simulink model "AC_base_1_VSM_1_22a"  (R2022a)
settings: Solver=ode3  StartTime=0.0  StopTime=8  FixedStep=HWSampleTime  RelTol=1e-3
undefined symbols (not defined in the file): ControlSampleTime, DiscIntNeverNeededParam, HWSampleTime, Ipwm_back, Ipwm_off, LCL, Manage, Oversample, Param, scaling_factor, SM, Ts, V_DC, VSMCTRL
libraries: fl_lib x51, nesl_utility x35, simulink x19, FriedrichLibrary x19, ee_lib x14, simulink_extras x7, TriphaseHardwaremodule x6, spsPower3phInstantaneousLib x1, spsEdgeDetectorLib x1, StateMachines x1, slpidlib x1
(part 1 of 4)
settings Model: Creator=e2n051  LastModifiedBy=e2n051

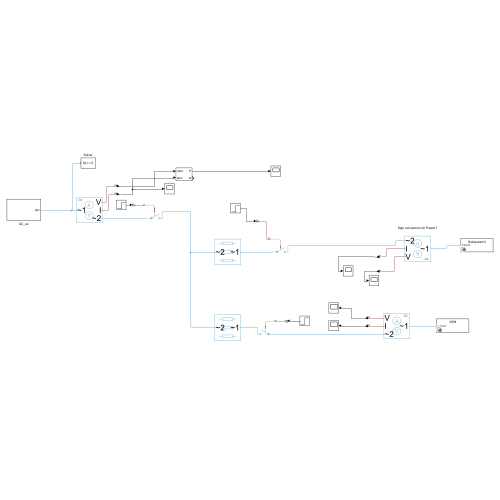
[thumbnail: Simulink's stored preview of the top-level diagram]
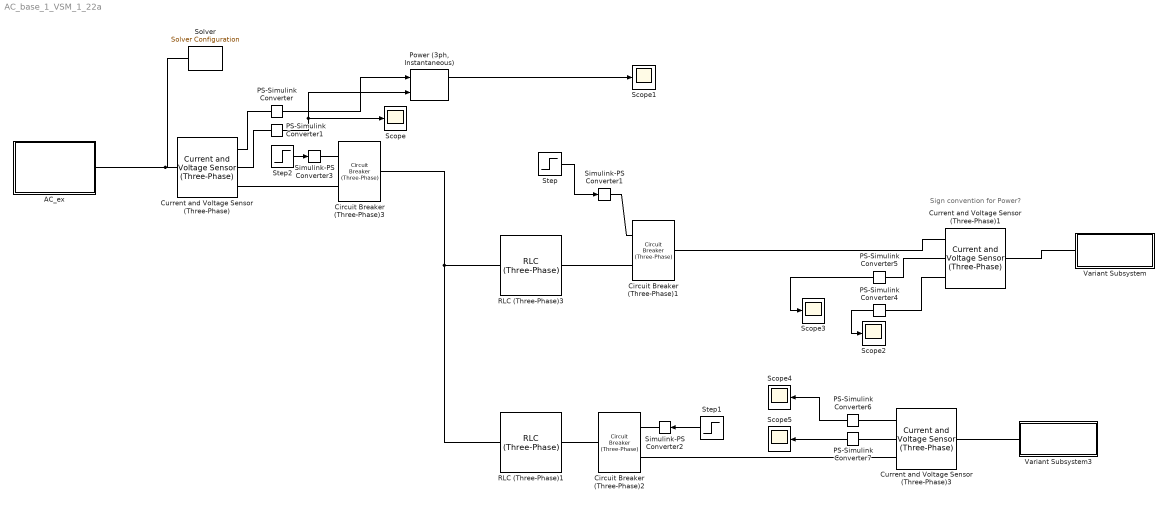
== system AC_base_1_VSM_1_22a ==
  note: Sign convention for Power?
  AC_ex : Subsystem
  Circuit Breaker (Three-Phase)1 : ee_lib/Switches & Breakers/Circuit Breaker (Three-Phase)  R_closed=0.001 Ohm  G_open=1e-6 1/Ohm  threshold=0.5 V  breaker_behavior=ee.enum.switches.breakerBehavior.zeroCrossingEnable
      settings: InternalSimscapePortConfiguration="{\"Bottom\":[],\"Left\":[{\"id\":\"vT\",\"label\":\"vT\",\"type\":\"input\"},{\"id\":\"N1\",\"label\":\"~1\",\"type\":\"foundation.electrical.three_phase\"}],\"Right\":[{\"id\":\"N2\",\"label\":\"~2\",\"type\":\"foundation.electrical.three_phase\"}],\"Top\":[]}"
  Circuit Breaker (Three-Phase)2 : ee_lib/Switches & Breakers/Circuit Breaker (Three-Phase)  R_closed=0.001 Ohm  G_open=1e-6 1/Ohm  threshold=0.5 V  breaker_behavior=ee.enum.switches.breakerBehavior.zeroCrossingEnable
      settings: InternalSimscapePortConfiguration="{\"Bottom\":[],\"Left\":[{\"id\":\"vT\",\"label\":\"vT\",\"type\":\"input\"},{\"id\":\"N1\",\"label\":\"~1\",\"type\":\"foundation.electrical.three_phase\"}],\"Right\":[{\"id\":\"N2\",\"label\":\"~2\",\"type\":\"foundation.electrical.three_phase\"}],\"Top\":[]}"
  Circuit Breaker (Three-Phase)3 : ee_lib/Switches & Breakers/Circuit Breaker (Three-Phase)  R_closed=0.001 Ohm  G_open=1e-6 1/Ohm  threshold=0.5 V  breaker_behavior=ee.enum.switches.breakerBehavior.zeroCrossingEnable
      settings: InternalSimscapePortConfiguration="{\"Bottom\":[],\"Left\":[{\"id\":\"vT\",\"label\":\"vT\",\"type\":\"input\"},{\"id\":\"N1\",\"label\":\"~1\",\"type\":\"foundation.electrical.three_phase\"}],\"Right\":[{\"id\":\"N2\",\"label\":\"~2\",\"type\":\"foundation.electrical.three_phase\"}],\"Top\":[]}"
  Current and Voltage Sensor (Three-Phase) : ee_lib/Sensors & Transducers/Current and Voltage Sensor (Three-Phase)  vMeasurementType=ee.enum.vmeasurement.lg  outputUnit=ee.enum.unit.si  SRated=100e6 A*V  VRated=24e3 V  I_specify=off  I_priority=None  I=[0, 0, 0] A  I_nominal_specify=off  I_nominal_value=1  I_nominal_unit=A  V_specify=off  V_priority=None  V=[0, 0, 0] V  V_nominal_specify=off  V_nominal_value=1  V_nominal_unit=V
      settings: InternalSimscapePortConfiguration="{\"Bottom\":[],\"Left\":[{\"id\":\"N1\",\"label\":\"~1\",\"type\":\"foundation.electrical.three_phase\"}],\"Right\":[{\"id\":\"V_output\",\"label\":\"V\",\"type\":\"output\"},{\"id\":\"I_output\",\"label\":\"I\",\"type\":\"output\"},{\"id\":\"N2\",\"label\":\"~2\",\"type\":\"foundation.electrical.three_phase\"}],\"Top\":[]}"
  Current and Voltage Sensor (Three-Phase)1 : ee_lib/Sensors & Transducers/Current and Voltage Sensor (Three-Phase)  vMeasurementType=ee.enum.vmeasurement.lg  outputUnit=ee.enum.unit.si  SRated=100e6 A*V  VRated=24e3 V  I_specify=off  I_priority=None  I=[0, 0, 0] A  I_nominal_specify=off  I_nominal_value=1  I_nominal_unit=A  V_specify=off  V_priority=None  V=[0, 0, 0] V  V_nominal_specify=off  V_nominal_value=1  V_nominal_unit=V
      settings: InternalSimscapePortConfiguration="{\"Bottom\":[],\"Left\":[{\"id\":\"N1\",\"label\":\"~1\",\"type\":\"foundation.electrical.three_phase\"}],\"Right\":[{\"id\":\"V_output\",\"label\":\"V\",\"type\":\"output\"},{\"id\":\"I_output\",\"label\":\"I\",\"type\":\"output\"},{\"id\":\"N2\",\"label\":\"~2\",\"type\":\"foundation.electrical.three_phase\"}],\"Top\":[]}"
  Current and Voltage Sensor (Three-Phase)3 : ee_lib/Sensors & Transducers/Current and Voltage Sensor (Three-Phase)  vMeasurementType=ee.enum.vmeasurement.lg  outputUnit=ee.enum.unit.si  SRated=100e6 A*V  VRated=24e3 V  I_specify=off  I_priority=None  I=[0, 0, 0] A  I_nominal_specify=off  I_nominal_value=1  I_nominal_unit=A  V_specify=off  V_priority=None  V=[0, 0, 0] V  V_nominal_specify=off  V_nominal_value=1  V_nominal_unit=V
      settings: InternalSimscapePortConfiguration="{\"Bottom\":[],\"Left\":[{\"id\":\"N1\",\"label\":\"~1\",\"type\":\"foundation.electrical.three_phase\"}],\"Right\":[{\"id\":\"V_output\",\"label\":\"V\",\"type\":\"output\"},{\"id\":\"I_output\",\"label\":\"I\",\"type\":\"output\"},{\"id\":\"N2\",\"label\":\"~2\",\"type\":\"foundation.electrical.three_phase\"}],\"Top\":[]}"
  PS-Simulink Converter{,1,4..7} (6 alike) : nesl_utility/PS-Simulink Converter  PhysicalDomain=network_engine_domain  SubClassName=ps_output  LeftPortType=input  RightPortType=output  PseudoPeriodic=off  Frequencies=[]  VectorFormat=inherit  Unit=inherit  AffineConversion=off
  "Power (3ph, Instantaneous)" : spsPower3phInstantaneousLib/Power (3ph, Instantaneous)
  RLC (Three-Phase)1 : ee_lib/Passive/RLC Assemblies/RLC (Three-Phase)  port_option=ee.enum.threePhasePort.composite  component_structure=ee.enum.rlc.structure.R  R=0.1 Ohm  L=1e-2 H  C=1e-6 F  R_parasitic=0 Ohm  G_parasitic=0 1/Ohm  IL_specify=off  IL_priority=High  IL=[0, 0, 0] A  IL_nominal_specify=off  IL_nominal_value=1  IL_nominal_unit=A  VC_specify=off  VC_priority=High  VC=[0, 0, 0] V  VC_nominal_specify=off  VC_nominal_value=1  VC_nominal_unit=V
      settings: InternalSimscapePortConfiguration="{\"Bottom\":[],\"Left\":[{\"id\":\"N1\",\"label\":\"~1\",\"type\":\"foundation.electrical.three_phase\"}],\"Right\":[{\"id\":\"N2\",\"label\":\"~2\",\"type\":\"foundation.electrical.three_phase\"}],\"Top\":[]}"
  RLC (Three-Phase)3 : ee_lib/Passive/RLC Assemblies/RLC (Three-Phase)  port_option=ee.enum.threePhasePort.composite  component_structure=ee.enum.rlc.structure.R  R=1 Ohm  L=1e-2 H  C=1e-6 F  R_parasitic=0 Ohm  G_parasitic=0 1/Ohm  IL_specify=off  IL_priority=High  IL=[0, 0, 0] A  IL_nominal_specify=off  IL_nominal_value=1  IL_nominal_unit=A  VC_specify=off  VC_priority=High  VC=[0, 0, 0] V  VC_nominal_specify=off  VC_nominal_value=1  VC_nominal_unit=V
      settings: InternalSimscapePortConfiguration="{\"Bottom\":[],\"Left\":[{\"id\":\"N1\",\"label\":\"~1\",\"type\":\"foundation.electrical.three_phase\"}],\"Right\":[{\"id\":\"N2\",\"label\":\"~2\",\"type\":\"foundation.electrical.three_phase\"}],\"Top\":[]}"
  Scope{,1..5} (6 alike) : Scope
  Simulink-PS Converter1 : nesl_utility/Simulink-PS Converter  PhysicalDomain=network_engine_domain  SubClassName=ps_input  LeftPortType=input  RightPortType=output  PseudoPeriodic=off  Frequencies=[]  NoiseDistribution=none  NoiseParameters=[]  Unit=1  AffineConversion=off  FilteringAndDerivatives=provide  SimscapeFilterOrder=1  InputFilterTimeConstant=0.001  UdotUserProvided=0
  Simulink-PS Converter2 : nesl_utility/Simulink-PS Converter  PhysicalDomain=network_engine_domain  SubClassName=ps_input  LeftPortType=input  RightPortType=output  PseudoPeriodic=off  Frequencies=[]  NoiseDistribution=none  NoiseParameters=[]  Unit=1  AffineConversion=off  FilteringAndDerivatives=provide  SimscapeFilterOrder=1  InputFilterTimeConstant=0.001  UdotUserProvided=0
  Simulink-PS Converter3 : nesl_utility/Simulink-PS Converter  PhysicalDomain=network_engine_domain  SubClassName=ps_input  LeftPortType=input  RightPortType=output  PseudoPeriodic=off  Frequencies=[]  NoiseDistribution=none  NoiseParameters=[]  Unit=1  AffineConversion=off  FilteringAndDerivatives=provide  SimscapeFilterOrder=1  InputFilterTimeConstant=0.001  UdotUserProvided=0
  Solver : nesl_utility/Solver Configuration  PhysicalDomain=network_engine_domain  SubClassName=solver  LeftPortType=input  RightPortType=generic  Tones=[]  Harmonics=[]  SimulateNoise=off  Profile=off  UseLocalSampling=off  EnableSwitchedLinearOptims=on  FrequencyDomain=off  UseCCode=off  RelTol=0.001  AbsTol=1e-06  MinStep=1e-09  ToWorkspace=off  RevertToSquareIcSolve=off  NumHomotopyIterations=100  PhasorMode=off  PhasorModeNumHarmonics=1  ConsistencySolver=NEWTON_FTOL  IndexReductionMethod=DerivativeReplacement  DoDC=off  ResidualTolerance=1e-2  ConsistencyTolSource=GLOBAL  ConsistencyAbsTol=0.001  ConsistencyRelTol=0.001  ConsistencyTolFactor=0.001  UseLocalSolver=on  LocalSolverChoice=NE_BACKWARD_EULER_ADVANCER  ResolveIndetEquations=on  FunctionEvalNumThread=1  LocalSolverSampleTime=HWSampleTime  DoFixedCost=off  MaxNonlinIter=3  MaxModeIter=2  ComputeImpulses=off  ImpulseIterations=2  LinearAlgebra=Sparse  LinearAlgebraNumThread=0  EquationFormulation=NE_TIME_EF  DelaysMemoryBudget=1024  AutomaticFiltering=on  FilteringTimeConstant=0.001  PartitionStorageMethod=AS_NEEDED  PartitionMemoryBudget=1024  PartitionMethod=FAST  MultibodyUseLocalSolver=off  MultibodyLocalSolverChoice=ODE1  MultibodyLocalSolverSampleTime=0.001
  Step : Step  After=0  SampleTime=0
  Step1 : Step  Time=0  After=0  SampleTime=0
  Step2 : Step  Time=6  SampleTime=0
  Variant Subsystem : Subsystem  Variant=on  VariantControlMode=label  LabelModeActiveChoice=Variant2  mask{VChoice=V2}
      mask prompts: VChoice "Select suystem"
      mask init:
      | choice = get_param(gcb,'VChoice');
      | vssBlk = gcb;
      | oldVariant = get_param(gcb,'LabelModeActiveChoice');
      | if strcmp(choice,'V1')
      |     
      |     set_param(vssBlk, 'LabelModeActiveChoice', 'Variant1');
      | else
      |     
      |     set_param(vssBlk, 'LabelModeActiveChoice', 'Variant2');
      | end
      mask TypeOptions VChoice: V1 | V2
  Variant Subsystem3 : Subsystem  Variant=on  VariantControlMode=label  LabelModeActiveChoice=Variant1  mask{VChoice=VSM}
      mask prompts: VChoice "Select suystem"
      mask init:
      | choice = get_param(gcb,'VChoice');
      | vssBlk = gcb;
      | oldVariant = get_param(gcb,'LabelModeActiveChoice');
      | if strcmp(choice,'VSM')
      |     
      |     set_param(vssBlk, 'LabelModeActiveChoice', 'Variant1');
      | else
      |     
      |     set_param(vssBlk, 'LabelModeActiveChoice', 'Variant2');
      | end
      mask TypeOptions VChoice: load | VSM
  wires:
  PS-Simulink Converter1/1 -> "Power (3ph, Instantaneous)"/2, Scope/1
  PS-Simulink Converter/1 -> "Power (3ph, Instantaneous)"/1
  "Power (3ph, Instantaneous)"/1 -> Scope1/1
  Step1/1 -> Simulink-PS Converter2/1
  PS-Simulink Converter6/1 -> Scope4/1
  PS-Simulink Converter7/1 -> Scope5/1
  Step/1 -> Simulink-PS Converter1/1
  PS-Simulink Converter4/1 -> Scope2/1
  PS-Simulink Converter5/1 -> Scope3/1
  Step2/1 -> Simulink-PS Converter3/1
  connections:
  PS-Simulink Converter1/LConn1 -- Current and Voltage Sensor (Three-Phase)/RConn2
  PS-Simulink Converter/LConn1 -- Current and Voltage Sensor (Three-Phase)/RConn1
  PS-Simulink Converter7/LConn1 -- Current and Voltage Sensor (Three-Phase)3/RConn2
  Circuit Breaker (Three-Phase)2/LConn1 -- Simulink-PS Converter2/RConn1
  Current and Voltage Sensor (Three-Phase)3/RConn1 -- PS-Simulink Converter6/LConn1
  RLC (Three-Phase)1/LConn1 -- Circuit Breaker (Three-Phase)2/RConn1
  RLC (Three-Phase)3/LConn1 -- Circuit Breaker (Three-Phase)1/LConn2
  RLC (Three-Phase)3/RConn1 -- RLC (Three-Phase)1/RConn1 -- Circuit Breaker (Three-Phase)3/RConn1
  Simulink-PS Converter1/RConn1 -- Circuit Breaker (Three-Phase)1/LConn1
  Variant Subsystem3/LConn1 -- Current and Voltage Sensor (Three-Phase)3/LConn1
  Current and Voltage Sensor (Three-Phase)/LConn1 -- Solver/RConn1 -- AC_ex/RConn1
  Circuit Breaker (Three-Phase)3/LConn2 -- Current and Voltage Sensor (Three-Phase)/RConn3
  Circuit Breaker (Three-Phase)2/LConn2 -- Current and Voltage Sensor (Three-Phase)3/RConn3
  Current and Voltage Sensor (Three-Phase)1/RConn1 -- PS-Simulink Converter4/LConn1
  Current and Voltage Sensor (Three-Phase)1/RConn2 -- PS-Simulink Converter5/LConn1
  Simulink-PS Converter3/RConn1 -- Circuit Breaker (Three-Phase)3/LConn1
  Current and Voltage Sensor (Three-Phase)1/LConn1 -- Variant Subsystem/LConn1
  Current and Voltage Sensor (Three-Phase)1/RConn3 -- Circuit Breaker (Three-Phase)1/RConn1

== system AC_base_1_VSM_1_22a/AC_ex ==
  Electrical Reference : fl_lib/Electrical/Electrical Elements/Electrical Reference
  Voltage Source (Three-Phase) : ee_lib/Sources/Voltage Source (Three-Phase)  vline_rms=sqrt(3) * 230 V  shift=0 deg  freq=50 Hz  impedance_option=1  SShortCircuit=1e6 A*V  XR=15  R=0.01 Ohm  L=3.97e-4 H  harmonic_option=0  harmonic_orders=[5, 7, 11, 13]  harmonic_ratios=[.1, .1, .1, .1]  G_parasitic=0 1/Ohm  I_specify=off  I_priority=None  I=[0, 0, 0] A  I_nominal_specify=off  I_nominal_value=1  I_nominal_unit=A
  abc : PMIOPort  Side=Right
  connections:
  abc/RConn1 -- Voltage Source (Three-Phase)/RConn1
  Voltage Source (Three-Phase)/LConn1 -- Electrical Reference/LConn1

== system AC_base_1_VSM_1_22a/Variant Subsystem ==
  note: 1) Add Subsystem or Model blocks as valid variant choices.
      | 2) You cannot connect blocks at this level. At simulation, connectivity is automatically
      | determined, based on the active variant and port name matching.
  Subsystem2 : Subsystem  VariantControl=Variant1
  Subsystem3 : Subsystem  VariantControl=Variant2
  Conn1 : PMIOPort  Side=Left

== system AC_base_1_VSM_1_22a/Variant Subsystem3 ==
  note: 1) Add Subsystem or Model blocks as valid variant choices.
      | 2) You cannot connect blocks at this level. At simulation, connectivity is automatically
      | determined, based on the active variant and port name matching.
  Subsystem3 : Subsystem  VariantControl=Variant2
  VSM : Subsystem  VariantControl=Variant1
  Conn1 : PMIOPort  Side=Left

== system AC_base_1_VSM_1_22a/Variant Subsystem/Subsystem2 ==
  Electrical Reference : fl_lib/Electrical/Electrical Elements/Electrical Reference
  Wye-Connected Load : ee_lib/Passive/RLC Assemblies/Wye-Connected Load  port_option=ee.enum.threePhasePort.composite  parameterization=ee.enum.rlc.parameterization.ratedpower  component_structure=ee.enum.rlc.structure.R  component_structure_PQ=ee.enum.rlc.structure.R  R=1 Ohm  L=1e-3 H  C=1e-6 F  VRated=230 V  FRated=60 Hz  P=1e3 W  Qpos=1e2 A*V  Qneg=-1e2 A*V  R_parasitic=0 Ohm  G_parasitic=0 1/Ohm  R_parasitic_PQ=0 Ohm  G_parasitic_PQ=0 1/Ohm  Vmag0=24e3 V  Vang0=0 deg  Freq0=60 Hz  IL_specify=off  IL_priority=High  IL=[0, 0, 0] A  IL_nominal_specify=off  IL_nominal_value=1  IL_nominal_unit=A  VC_specify=off  VC_priority=High  VC=[0, 0, 0] V  VC_nominal_specify=off  VC_nominal_value=1  VC_nominal_unit=V
  Conn1 : PMIOPort  Side=Left
  connections:
  Wye-Connected Load/LConn1 -- Conn1/RConn1
  Electrical Reference/LConn1 -- Wye-Connected Load/RConn1

== system AC_base_1_VSM_1_22a/Variant Subsystem/Subsystem3 ==
  Delta-Connected Load1 : ee_lib/Passive/RLC Assemblies/Delta-Connected Load  port_option=ee.enum.threePhasePort.composite  parameterization=ee.enum.rlc.parameterization.ratedpower  component_structure=ee.enum.rlc.structure.R  component_structure_PQ=ee.enum.rlc.structure.R  R=1 Ohm  L=1e-3 H  C=1e-6 F  VRated=230 V  FRated=60 Hz  P=3000 W  Qpos=1e2 A*V  Qneg=-1e2 A*V  R_parasitic=0 Ohm  G_parasitic=0 1/Ohm  R_parasitic_PQ=0 Ohm  G_parasitic_PQ=0 1/Ohm  Vmag0=24e3 V  Vang0=0 deg  Freq0=60 Hz  IL_specify=off  IL_priority=High  IL=[0, 0, 0] A  IL_nominal_specify=off  IL_nominal_value=1  IL_nominal_unit=A  VC_specify=off  VC_priority=High  VC=[0, 0, 0] V  VC_nominal_specify=off  VC_nominal_value=1  VC_nominal_unit=V
      settings: InternalSimscapePortConfiguration="{\"Bottom\":[],\"Left\":[{\"id\":\"N\",\"label\":\"~\",\"type\":\"foundation.electrical.three_phase\"}],\"Right\":[],\"Top\":[]}"
  Conn1 : PMIOPort  Side=Left
  connections:
  Delta-Connected Load1/LConn1 -- Conn1/RConn1

== system AC_base_1_VSM_1_22a/Variant Subsystem3/Subsystem3 ==
  Delta-Connected Load1 : ee_lib/Passive/RLC Assemblies/Delta-Connected Load  port_option=ee.enum.threePhasePort.composite  parameterization=ee.enum.rlc.parameterization.ratedpower  component_structure=ee.enum.rlc.structure.R  component_structure_PQ=ee.enum.rlc.structure.R  R=1 Ohm  L=1e-3 H  C=1e-6 F  VRated=230 V  FRated=60 Hz  P=300 W  Qpos=1e2 A*V  Qneg=-1e2 A*V  R_parasitic=0 Ohm  G_parasitic=0 1/Ohm  R_parasitic_PQ=0 Ohm  G_parasitic_PQ=0 1/Ohm  Vmag0=24e3 V  Vang0=0 deg  Freq0=60 Hz  IL_specify=off  IL_priority=High  IL=[0, 0, 0] A  IL_nominal_specify=off  IL_nominal_value=1  IL_nominal_unit=A  VC_specify=off  VC_priority=High  VC=[0, 0, 0] V  VC_nominal_specify=off  VC_nominal_value=1  VC_nominal_unit=V
      settings: InternalSimscapePortConfiguration="{\"Bottom\":[],\"Left\":[{\"id\":\"N\",\"label\":\"~\",\"type\":\"foundation.electrical.three_phase\"}],\"Right\":[],\"Top\":[]}"
  Conn1 : PMIOPort  Side=Left
  connections:
  Delta-Connected Load1/LConn1 -- Conn1/RConn1

== system AC_base_1_VSM_1_22a/Variant Subsystem3/VSM ==
  ADC-Emulator_F : Subsystem  AncestorBlock=TriphaseHardwaremodule/ADC-Emulator_F  mask{ADC_Emulation=off, ControlSampleTime=ControlSampleTime, HWSampleTime=HWSampleTime, Vac_max=1000, Vac_bit=16, Iac_max=400, Iac_bit=16, Vdc_max=1000, Vdc_bit=16}
      mask prompts: Vac_max "AC Voltage Range"; Vac_bit "ADC resolution [bit]"; Iac_max "AC Current Range"; Iac_bit "ADC resolution [bit]"; Vdc_max "DC Voltage Range"; Vdc_bit "ADC resolution [bit]"
      mask init:
      | ParamValue=get_param(gcb,'ADC_Emulation');
      | set_param([gcb '/adc_i_inverter'],'ADC_Emulation',ParamValue);
      | set_param([gcb '/adc_i_out'],'ADC_Emulation',ParamValue);
      | set_param([gcb '/adc_u_cap'],'ADC_Emulation',ParamValue);
      | set_param([gcb '/adc_u_dc'],'ADC_Emulation',ParamValue);
      | set_param([gcb '/adc_u_out'],'ADC_Emulation',ParamValue);
      mask TypeOptions ADC_Emulation: off | on
      mask DialogControl GrpADC Prompt: ADC-Emulation
      mask DialogControl ADC_Text Prompt: ADC-emulation emulates the quantization resulting from AD-conversion. Moving Average is always applied over one ControlSampleTime
  Bus Selector : BusSelector  OutputSignals=meas_i_inverter,meas_i_out
  Electrical Reference : fl_lib/Electrical/Electrical Elements/Electrical Reference
  Inverter AverageMdl LC SimScape2 : Subsystem  VariantControl=PMXXF33C  mask{L1=LCL.SI.L1, R_L1=LCL.SI.R1, C1=LCL.SI.C, R_C1=LCL.SI.Rc}
      mask prompts: L1 "Inductance L1 [H]"; R_L1 "Resistance of L1 [Ohm]"; C1 "Capacitance C1 [F]"; R_C1 "Parallel resistance of C1 [Ohm]"
      mask DialogControl GrpLC Prompt: LC(L)(C)-Filter
  Scope : Scope  NumInputPorts=2
  VSM1 : Subsystem
  Conn1 : PMIOPort  Side=Left
  wires:
  Bus Selector/2 -> Scope/2  "<meas_i_out>"
  Bus Selector/1 -> Scope/1  "<meas_i_inverter>"
  VSM1/1(Ctrl) -> Inverter AverageMdl LC SimScape2/1(Setpoints)
  Inverter AverageMdl LC SimScape2/1(Measurements) -> ADC-Emulator_F/1(meas)
  Inverter AverageMdl LC SimScape2/2(measf) -> Bus Selector/1
  ADC-Emulator_F/1(measOut) -> VSM1/1(Measurement)
  connections:
  Inverter AverageMdl LC SimScape2/RConn2 -- Electrical Reference/LConn1
  Conn1/RConn1 -- Inverter AverageMdl LC SimScape2/RConn1

== system AC_base_1_VSM_1_22a/Variant Subsystem3/VSM/ADC-Emulator_F ==
  meas : Inport
  Bus Creator : BusCreator  Inputs=8
  Bus Selector : BusSelector  OutputSignals=Inv1.meas_u_dc,Inv1.meas_u_cap,Inv1.meas_u_out,Inv1.meas_i_inverter,Inv1.meas_i_out,Inv1.connection_state,Inv1.enabled
  Constant : Constant  Value=[1 1 1]
  Rate Transition : RateTransition  Integrity=off  InitialCondition=-1  OutPortSampleTime=ControlSampleTime
  Rate Transition1 : RateTransition  Integrity=off  InitialCondition=-1  OutPortSampleTime=ControlSampleTime
  adc_i_inverter : TriphaseHardwaremodule/adc  ADC_Emulation=off  ControlSampleTime=ControlSampleTime  HWSampleTime=HWSampleTime  MeasMax=Iac_max  MeasBits=Iac_bit
  adc_i_out : TriphaseHardwaremodule/adc  ADC_Emulation=off  ControlSampleTime=ControlSampleTime  HWSampleTime=HWSampleTime  MeasMax=Iac_max  MeasBits=Iac_bit
  adc_u_cap : TriphaseHardwaremodule/adc  ADC_Emulation=off  ControlSampleTime=ControlSampleTime  HWSampleTime=HWSampleTime  MeasMax=Vac_max  MeasBits=Vac_bit
  adc_u_dc : TriphaseHardwaremodule/adc  ADC_Emulation=off  ControlSampleTime=ControlSampleTime  HWSampleTime=HWSampleTime  MeasMax=Vdc_max  MeasBits=Vdc_bit
  adc_u_inverter : TriphaseHardwaremodule/adc  ADC_Emulation=off  ControlSampleTime=ControlSampleTime  HWSampleTime=HWSampleTime  MeasMax=Vac_max  MeasBits=Vac_bit
  adc_u_out : TriphaseHardwaremodule/adc  ADC_Emulation=off  ControlSampleTime=ControlSampleTime  HWSampleTime=HWSampleTime  MeasMax=Vac_max  MeasBits=Vac_bit
  measOut : Outport  VectorParamsAs1DForOutWhenUnconnected=off
  wires:
  Bus Selector/1 -> adc_u_dc/1  "<meas_u_dc>"
  Rate Transition1/1 -> Bus Creator/8  "enabled"
  Rate Transition/1 -> Bus Creator/7  "connection_state"
  adc_u_cap/1 -> Bus Creator/3  "meas_u_cap"
  Bus Creator/1 -> measOut/1
  adc_u_out/1 -> Bus Creator/4  "meas_u_out"
  adc_i_out/1 -> Bus Creator/6  "meas_i_out"
  adc_i_inverter/1 -> Bus Creator/5  "meas_i_inverter"
  adc_u_dc/1 -> Bus Creator/1  "meas_u_dc"
  meas/1 -> Bus Selector/1
  adc_u_inverter/1 -> Bus Creator/2  "meas_u_inverter"
  Bus Selector/7 -> Rate Transition1/1  "<enabled>"
  Bus Selector/6 -> Rate Transition/1  "<connection_state>"
  Bus Selector/5 -> adc_i_out/1  "<meas_i_out>"
  Bus Selector/4 -> adc_i_inverter/1  "<meas_i_inverter>"
  Bus Selector/3 -> adc_u_out/1  "<meas_u_out>"
  Bus Selector/2 -> adc_u_cap/1  "<meas_u_cap>"
  Constant/1 -> adc_u_inverter/1

== system AC_base_1_VSM_1_22a/Variant Subsystem3/VSM/Inverter AverageMdl LC SimScape2 ==
  Setpoints : Inport
  Bus Creator : BusCreator  Inputs=1
  Bus Creator1 : BusCreator  Inputs=5
  Bus Selector : BusSelector  OutputSignals=meas_u_cap,meas_u_out,meas_i_inverter,meas_i_out,block
  Modul F30 fixed DC voltage Average SimScape : Subsystem  mask{L1=L1, R_L1=R_L1, C1=C1, R_C1=R_C1}
      mask prompts: L1 "Inductance L1 [H]"; R_L1 "Resistance of L1 [Ohm]"; C1 "Capacitance C1 [F]"; R_C1 "Parallel resistance of C1 [Ohm]"
      mask DialogControl GrpLoad Prompt: Triphase
      mask DialogControl LC Prompt: LC(L)(C)
      mask DialogControl GrpLC Prompt: LC(L)(C)-Filter
  ABC : PMIOPort  Side=Right
  N : PMIOPort  Port=2  Side=Right
  Measurements : Outport  VectorParamsAs1DForOutWhenUnconnected=off
  measf : Outport  Port=2  VectorParamsAs1DForOutWhenUnconnected=off
  wires:
  Modul F30 fixed DC voltage Average SimScape/1(meas) -> Bus Creator/1  "Inv1"
  Bus Creator/1 -> Measurements/1
  Setpoints/1 -> Modul F30 fixed DC voltage Average SimScape/1(ctrl)
  Modul F30 fixed DC voltage Average SimScape/2(measf) -> Bus Selector/1
  Bus Selector/1 -> Bus Creator1/1  "<meas_u_cap>"
  Bus Selector/2 -> Bus Creator1/2  "<meas_u_out>"
  Bus Selector/3 -> Bus Creator1/3  "<meas_i_inverter>"
  Bus Selector/4 -> Bus Creator1/4  "<meas_i_out>"
  Bus Creator1/1 -> measf/1
  Bus Selector/5 -> Bus Creator1/5  "<block>"
  connections:
  N/RConn1 -- Modul F30 fixed DC voltage Average SimScape/LConn1
  ABC/RConn1 -- Modul F30 fixed DC voltage Average SimScape/RConn1

== system AC_base_1_VSM_1_22a/Variant Subsystem3/VSM/VSM1 ==
  Measurement : Inport
  Bus Selector : BusSelector  OutputSignals=connected,enabled
  Bus Creator6 : BusCreator  Inputs=3  OutDataTypeStr=Bus: FeedbackDCBus
  Constant1 : Constant  SampleTime=SM.TsTimer
  Constant3 : Constant  SampleTime=SM.TsTimer
  Constant4 : Constant  SampleTime=SM.TsTimer
  Display : Display
  Display1 : Display
  MeasInv1 : Subsystem  Commented=on
      settings: OpenFcn=open_system(find_system(gcb,'BlockType','Scope'))
  Terminator : Terminator
  Unit Delay : UnitDelay  SampleTime=ControlSampleTime  HasFrameUpgradeWarning=on
  VSM : Subsystem  AncestorBlock=ControLibrary/VSM  ClipboardFcn=createTriphaseBus  mask{Ctrl=VSMCTRL, pu=VSMCTRL.PU, DoN=off}
      mask prompts: Ctrl "ParamStruct"; pu "PU-System"; DoN "N Leiter Schalten (4 Phasen)"
      mask init:
      | if DoN
      |     NrChannels=4;
      | else
      |     NrChannels=3;
      | end
  command_center : Subsystem
  diagPlot : Subsystem
  Ctrl : Outport  VectorParamsAs1DForOutWhenUnconnected=off
  wires:
  Measurement/1 -> VSM/2(meas), MeasInv1/1(SimOut)
  VSM/3(diag) -> diagPlot/1(Diag)  "Inv1"
  VSM/1(ctrl) -> Unit Delay/1  "Inv1"
  VSM/2(feedback) -> Bus Selector/1, command_center/1(Feed_AC)
  command_center/2(cmd_ac) -> VSM/1(cmd)
  Bus Selector/1 -> Display/1  "<connected>"
  Bus Selector/2 -> Display1/1  "<enabled>"
  command_center/1(cmd_tp) -> Terminator/1
  Constant4/1 -> Bus Creator6/2  "enabled"
  Bus Creator6/1 -> command_center/2(Feed_DC)
  Constant3/1 -> Bus Creator6/1  "connected"
  Constant1/1 -> Bus Creator6/3  "DCBus_isset"
  Unit Delay/1 -> Ctrl/1

== system AC_base_1_VSM_1_22a/Variant Subsystem3/VSM/Inverter AverageMdl LC SimScape2/Modul F30 fixed DC voltage Average SimScape ==
  ctrl : Inport
  Bus Selector : BusSelector  OutputSignals=connect
  Phase Splitter : ee_lib/Connectors & References/Phase Splitter
  Rate Transition1 : RateTransition  Commented=on  Integrity=off  InitialCondition=-1  OutPortSampleTime=ControlSampleTime
  S_connect : ee_lib/Switches & Breakers/SPST Switch (Three-Phase)  R_closed=1e-9 Ohm  G_open=1e-6 1/Ohm  threshold=0.5 V  i_vT_specify=off  i_vT_priority=None  i_vT=0 A  i_vT_nominal_specify=off  i_vT_nominal_value=1  i_vT_nominal_unit=A  I_specify=off  I_priority=None  I=[ 0 0 0 ] A  I_nominal_specify=off  I_nominal_value=1  I_nominal_unit=A  V_specify=off  V_priority=None  V=[ 0 0 0 ] V  V_nominal_specify=off  V_nominal_value=1  V_nominal_unit=V  i_a_specify=off  i_a_priority=None  i_a=0 A  i_a_nominal_specify=off  i_a_nominal_value=1  i_a_nominal_unit=A  v_a_specify=off  v_a_priority=None  v_a=0 V  v_a_nominal_specify=off  v_a_nominal_value=1  v_a_nominal_unit=V  i_b_specify=off  i_b_priority=None  i_b=0 A  i_b_nominal_specify=off  i_b_nominal_value=1  i_b_nominal_unit=A  v_b_specify=off  v_b_priority=None  v_b=0 V  v_b_nominal_specify=off  v_b_nominal_value=1  v_b_nominal_unit=V  i_c_specify=off  i_c_priority=None  i_c=0 A  i_c_nominal_specify=off  i_c_nominal_value=1  i_c_nominal_unit=A  v_c_specify=off  v_c_priority=None  v_c=0 V  v_c_nominal_specify=off  v_c_nominal_value=1  v_c_nominal_unit=V
      settings: InternalSimscapePortConfiguration="{\"Bottom\":[],\"Left\":[{\"id\":\"vT\",\"label\":\"vT\",\"type\":\"input\"},{\"id\":\"N1\",\"label\":\"~1\",\"type\":\"foundation.electrical.three_phase\"}],\"Right\":[{\"id\":\"N2\",\"label\":\"~2\",\"type\":\"foundation.electrical.three_phase\"}],\"Top\":[]}"
  Simulink-PS Converter : nesl_utility/Simulink-PS Converter  PhysicalDomain=network_engine_domain  SubClassName=ps_input  LeftPortType=input  RightPortType=output  PseudoPeriodic=off  Frequencies=[]  NoiseDistribution=none  NoiseParameters=[]  Unit=1  AffineConversion=off  FilteringAndDerivatives=zero  SimscapeFilterOrder=1  InputFilterTimeConstant=0.001  UdotUserProvided=1
  ctrlSelect3 : Subsystem
  measMerge3 : Subsystem
  simscape_bridgefilter_aca : Subsystem  mask{L1=L1, R_L1=R_L1, C1=C1, R_C1=R_C1}
      mask prompts: L1 "Inductance L1 [H]"; R_L1 "Resistance of L1 [Ohm]"; C1 "Capacitance C1 [F]"; R_C1 "Parallel resistance of C1 [Ohm]"
      mask DialogControl LC Prompt: LC(L)(C)
      mask DialogControl GrpLC Prompt: LC(L)(C)-Filter
  simscape_bridgefilter_aca1 : Subsystem  mask{L1=L1, R_L1=R_L1, C1=C1, R_C1=R_C1}
      mask prompts: L1 "Inductance L1 [H]"; R_L1 "Resistance of L1 [Ohm]"; C1 "Capacitance C1 [F]"; R_C1 "Parallel resistance of C1 [Ohm]"
      mask DialogControl LC Prompt: LC(L)(C)
      mask DialogControl GrpLC Prompt: LC(L)(C)-Filter
  simscape_bridgefilter_aca2 : Subsystem  mask{L1=L1, R_L1=R_L1, C1=C1, R_C1=R_C1}
      mask prompts: L1 "Inductance L1 [H]"; R_L1 "Resistance of L1 [Ohm]"; C1 "Capacitance C1 [F]"; R_C1 "Parallel resistance of C1 [Ohm]"
      mask DialogControl LC Prompt: LC(L)(C)
      mask DialogControl GrpLC Prompt: LC(L)(C)-Filter
  N : PMIOPort  Side=Left
  ABC : PMIOPort  Port=2  Side=Right
  meas : Outport  VectorParamsAs1DForOutWhenUnconnected=off
  measf : Outport  Port=2  VectorParamsAs1DForOutWhenUnconnected=off
  wires:
  ctrlSelect3/1(ctrl1) -> Bus Selector/1, simscape_bridgefilter_aca/1(ctrl)
  [ctrl3] -> simscape_bridgefilter_aca2/1(ctrl)
  [ctrl2] -> simscape_bridgefilter_aca1/1(ctrl)
  ctrlSelect3/2(ctrl2) -> [ctrl2]
  ctrlSelect3/3(ctrl3) -> [ctrl3]
  ctrl/1 -> ctrlSelect3/1(ctrl)
  [meas2] -> measMerge3/2(meas2)
  simscape_bridgefilter_aca2/1(meas) -> [meas3]
  simscape_bridgefilter_aca1/1(meas) -> [meas2]
  [meas3] -> measMerge3/3(meas3)
  simscape_bridgefilter_aca/1(meas) -> measMerge3/1(meas1)
  measMerge3/1(meas) -> meas/1, measf/1
  Bus Selector/1 -> [connect]  "<connect>"
  [connect] -> Simulink-PS Converter/1
  connections:
  simscape_bridgefilter_aca/LConn2 -- simscape_bridgefilter_aca1/LConn2 -- simscape_bridgefilter_aca2/LConn2 -- N/RConn1
  simscape_bridgefilter_aca/RConn1 -- simscape_bridgefilter_aca2/RConn1 -- simscape_bridgefilter_aca1/RConn1
  simscape_bridgefilter_aca2/LConn1 -- Phase Splitter/RConn3
  Phase Splitter/RConn1 -- simscape_bridgefilter_aca/LConn1
  simscape_bridgefilter_aca1/LConn1 -- Phase Splitter/RConn2
  Simulink-PS Converter/RConn1 -- S_connect/LConn1
  S_connect/LConn2 -- ABC/RConn1
  S_connect/RConn1 -- Phase Splitter/LConn1

== system AC_base_1_VSM_1_22a/Variant Subsystem3/VSM/VSM1/MeasInv1 ==
  SimOut : Inport
  Bus Selector1 : BusSelector  OutputSignals=meas_u_dc,meas_u_cap,meas_u_out,meas_i_inverter,meas_i_out,connection_state,enabled
  Meas_Inv1 : Scope  NumInputPorts=7
  To Workspace1 : ToWorkspace  VariableName=MeasAC_Ucap  SampleTime=-1
  To Workspace2 : ToWorkspace  VariableName=MeasAC_Uout  SampleTime=-1
  To Workspace3 : ToWorkspace  VariableName=MeasAC_Iinv  SampleTime=-1
  To Workspace4 : ToWorkspace  VariableName=MeasAC_Iout  SampleTime=-1
  To Workspace7 : ToWorkspace  VariableName=MeasAC_Udc  SampleTime=-1
  wires:
  Bus Selector1/7 -> Meas_Inv1/7  "<enabled>"
  Bus Selector1/6 -> Meas_Inv1/6  "<connection_state>"
  Bus Selector1/5 -> To Workspace4/1, Meas_Inv1/5  "<meas_i_out>"
  Bus Selector1/4 -> To Workspace3/1, Meas_Inv1/4  "<meas_i_inverter>"
  Bus Selector1/3 -> To Workspace2/1, Meas_Inv1/3  "<meas_u_out>"
  Bus Selector1/2 -> To Workspace1/1, Meas_Inv1/2  "<meas_u_cap>"
  Bus Selector1/1 -> To Workspace7/1, Meas_Inv1/1  "<meas_u_dc>"
  SimOut/1 -> Bus Selector1/1

== system AC_base_1_VSM_1_22a/Variant Subsystem3/VSM/VSM1/VSM ==
  cmd : Inport
  meas : Inport  Port=2
  BUS_GENERATION : Subsystem
  CONTROL : Subsystem
  MANAGEMENT : Subsystem  mask(VSMCC Management){Mgn=Ctrl.Mgn}
      mask prompts: Mgn "Mgn Parameters"
      mask help:
      | Mgn(.PQSpRateUp, .PQSpRateDown, PQSpMax, .PQSpMin)
      |
      | Parameter nicht auf der Maske:
      | ControlSampleTime
  Meas : Subsystem  mask(Messeinrichtung für VSM mit CC){PU=pu, PLL=Ctrl.PLL}
      mask prompts: PU "PU System"; PLL "PLL Parameters"
      mask help:
      | PU System(.Vb, .Ib)
      |
      | PLL Parameter (.kp, .ki)
      |
      | Parameter nicht auf der Maske:
      | NrChannels
      | ControlSampleTime
  ctrl : Outport  VectorParamsAs1DForOutWhenUnconnected=off  LockScale=on
  feedback : Outport  Port=2  VectorParamsAs1DForOutWhenUnconnected=off
  diag : Outport  Port=3  VectorParamsAs1DForOutWhenUnconnected=off
  wires:
  meas/1 -> Meas/1(MEASIN)
  cmd/1 -> MANAGEMENT/1(CMD)
  CONTROL/1(CONTROL) -> Meas/2("CONTROL "), BUS_GENERATION/2(CONTROL)
  BUS_GENERATION/1(ctrl) -> ctrl/1
  BUS_GENERATION/2(feedback) -> feedback/1
  CONTROL/2(diagCtrl) -> diag/1
  MANAGEMENT/1(MANAGE) -> CONTROL/1(MANAGE), BUS_GENERATION/1(MANAGE)
  Meas/1(MEAS) -> CONTROL/2(MEAS), MANAGEMENT/2(MEAS)

== system AC_base_1_VSM_1_22a/Variant Subsystem3/VSM/VSM1/command_center ==
  note: State Machine for TP <-> WP SIM
      |
      | State Index:
      | 0: Error
      | 1: Stop
      | 2: Ready (Precharge, Connected + Enable DC)
      | 3: Connect AC
      | 4: Enable AC
  Feed_AC : Inport
  Feed_DC : Inport  Port=2
  Bus Assignment : BusAssignment  AssignedSignals=Manage.connect,Manage.enable,Param.VSM.sp_PQ,Param.VSM.sp_E
  Bus Selector2 : BusSelector  OutputSignals=connect,enable
  Bus Creator1 : BusCreator  Inputs=2
  Constant : Constant
  Display1 : Display
  Display2 : Display
  Display5 : Display
  Error ACK : Subsystem
      settings: OpenFcn=|
      | switch get_param([gcb '/Toggle'],'Value')
      |     case '1'
      |         set_param([gcb '/Toggle'],'Value', '0');
      |         set_param(gcb,'BackgroundColor','[0.8500    0.3250    0.0980]');
      |     case '0'
      |         set_param([gcb '/Toggle'],'Value', '1');
      |         set_param(gcb,'BackgroundColor','[0.4660    0.6740    0.1880]');
      | end
      mask Display: port_label('output',1,'')
  Rate Transition3 : RateTransition  Integrity=off  OutPortSampleTime=ControlSampleTime
  Shortcut1 : Subsystem  mask{path=./ControlLibrary/FriedrichLibrary.slx}
      settings: OpenFcn=findsimscopes
      mask Display: disp('Open Scopes...')
  Step3 : Step  Time=5.0+100  Before=[0.5 0]*-1  After=[0.1 0]  SampleTime=0
  Step4 : Step  Time=0  SampleTime=0
  Subsystem : Subsystem
  cmd_VSM : Subsystem  AncestorBlock=ControLibrary/cmd_VSM template
  cmd_tp : Outport  VectorParamsAs1DForOutWhenUnconnected=off
  cmd_ac : Outport  Port=2  VectorParamsAs1DForOutWhenUnconnected=off
  wires:
  Rate Transition3/1 -> cmd_ac/1
  cmd_VSM/1(cmd_ac) -> Bus Assignment/1
  Bus Assignment/1 -> Rate Transition3/1
  Error ACK/1(Out) -> Bus Creator1/1  "error_ack"
  Bus Creator1/1 -> cmd_tp/1
  Bus Selector2/1 -> Display1/1, Bus Assignment/2  "<connect>"
  Bus Selector2/2 -> Display2/1, Bus Assignment/3  "<enable>"
  Subsystem/1(precharge) -> Bus Creator1/2, Display5/1
  Feed_AC/1 -> Subsystem/1(In1)
  Feed_DC/1 -> Subsystem/2(In2)
  Subsystem/2(cmd_ac) -> Bus Selector2/1
  Step4/1 -> Subsystem/Enable
  Step3/1 -> Bus Assignment/4
  Constant/1 -> Bus Assignment/5

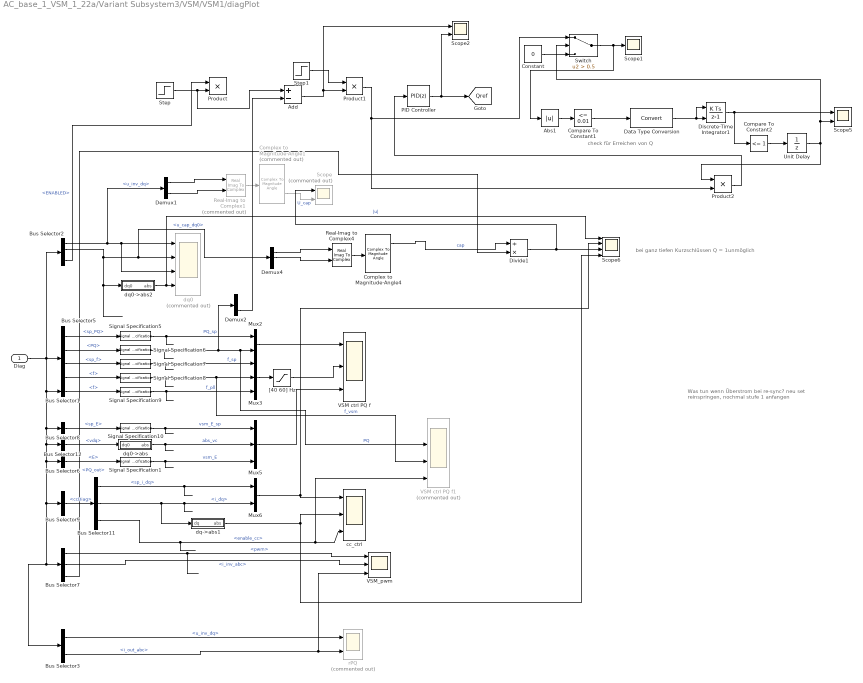
== system AC_base_1_VSM_1_22a/Variant Subsystem3/VSM/VSM1/diagPlot ==
  note: Was tun wenn Überstrom bei re-sync?
      |
      | neu set reinspringen, nochmal stufe 1 anfangen
  note: bei ganz tiefen Kurzschlüssen Q = 1unmöglich
  note: check für Erreichen von Q
  Diag : Inport
  Abs1 : Abs  SaturateOnIntegerOverflow=off
  Add : Sum  Inputs=+-
  Bus Selector1 : BusSelector  OutputSignals=measDiag.PLL.f
  Bus Selector11 : BusSelector  OutputSignals=sp_i_dq,i_dq,enable_cc
  Bus Selector12 : BusSelector  OutputSignals=measDiag.PLL.vdq
  Bus Selector2 : BusSelector  OutputSignals=u_inv_dq,measDiag.u_cap.u_cap_dq0,measDiag.u_cap.u_cap_abc,manage.ENABLED
  Bus Selector3 : BusSelector  OutputSignals=u_inv_dq,measDiag.i_out.i_out_abc
  Bus Selector5 : BusSelector  OutputSignals=manage.sp_VSM.sp_PQ,measDiag.PQ,manage.sp_VSM.sp_f,vsmDiag.f
  Bus Selector6 : BusSelector  OutputSignals=vsmDiag.E
  Bus Selector7 : BusSelector  OutputSignals=pwmDiag.pwm,measDiag.i_inv.i_inv_abc,measDiag.PQ_out
  Bus Selector8 : BusSelector  OutputSignals=vsmDiag.sp_VSM.sp_E
  Bus Selector9 : BusSelector  OutputSignals=ccDiag
  Compare To Constant1 : simulink/Logic and Bit Operations/Compare To Constant  relop=<=  const=0.01  OutDataTypeStr=boolean
  Compare To Constant2 : simulink/Logic and Bit Operations/Compare To Constant  relop=<=  const=1  OutDataTypeStr=boolean
  Complex to Magnitude-Angle1 : ComplexToMagnitudeAngle  Commented=on
  Complex to Magnitude-Angle4 : ComplexToMagnitudeAngle
  Constant : Constant  Value=0
  Data Type Conversion : DataTypeConversion  SaturateOnIntegerOverflow=off  RndMeth=Floor
  Demux1 : Demux  Outputs=2
  Demux2 : Demux  Outputs=2
  Demux4 : Demux  Outputs=3
  Discrete-Time Integrator1 : DiscreteIntegrator  ExternalReset=rising  SampleTime=-1  ICPrevOutput=DiscIntNeverNeededParam  ICPrevScaledInput=DiscIntNeverNeededParam
  Divide1 : Product  Inputs=/*
  Mux2 : Mux  Inputs=2
  Mux3 : Mux  Inputs=3
  Mux5 : Mux  Inputs=3
  Mux6 : Mux  Inputs=2
  PID Controller : slpidlib/PID Controller  Controller=PID  Form=Parallel  TimeDomain=Discrete-time  UseExternalTs=off  SampleTime=-1  IntegratorMethod=Forward Euler  FilterMethod=Forward Euler  ControllerParametersSource=internal  P=0.1  I=1  UseKiTs=off  D=0  N=100  UseFilter=on  TunerSelectOption=Transfer Function Based (PID Tuner App)  InitialConditionSource=internal  InitialConditionForIntegrator=1  InitialConditionForFilter=0  DifferentiatorICPrevScaledInput=0  ExternalReset=none  TrackingMode=off  Kt=1  LimitOutput=off  SatLimitsSource=internal  UpperSaturationLimit=inf  LowerSaturationLimit=-inf  LinearizeAsGain=on  AntiWindupMode=none  Kb=1  POutMin=[]  POutMax=[]  IOutMin=[]  IOutMax=[]  DOutMin=[]  DOutMax=[]  NOutMin=[]  NOutMax=[]  SumOutMin=[]  SumOutMax=[]  SaturationOutMin=[]  SaturationOutMax=[]  PParamMin=[]  PParamMax=[]  IParamMin=[]  IParamMax=[]  DParamMin=[]  DParamMax=[]  NParamMin=[]  NParamMax=[]  KbParamMin=[]  KbParamMax=[]  KtParamMin=[]  KtParamMax=[]  KbOutMin=[]  KbOutMax=[]  KtOutMin=[]  KtOutMax=[]  IntegratorOutMin=[]  IntegratorOutMax=[]  FilterOutMin=[]  FilterOutMax=[]  SumI1OutMin=[]  SumI1OutMax=[]  SumI2OutMin=[]  SumI2OutMax=[]  SumI3OutMin=[]  SumI3OutMax=[]  SumI4OutMin=[]  SumI4OutMax=[]  SumDOutMin=[]  SumDOutMax=[]  DifferentiatorOutMin=[]  DifferentiatorOutMax=[]  FilterDiffOutCoefMin=[]  FilterDiffOutCoefMax=[]  ReciprocalOutMin=[]  ReciprocalOutMax=[]  SumDenOutMin=[]  SumDenOutMax=[]  SumNumOutMin=[]  SumNumOutMax=[]  DivideOutMin=[]  DivideOutMax=[]  UdiffTsProdOutMin=[]  UdiffTsProdOutMax=[]  NTsProdOutMin=[]  NTsProdOutMax=[]  UintegralTsProdOutMin=[]  UintegralTsProdOutMax=[]  UngainTsProdOutMin=[]  UngainTsProdOutMax=[]  IntegratorContinuousStateAttributes=''  IntegratorStateMustResolveToSignalObject=off  IntegratorRTWStateStorageClass=Auto  FilterContinuousStateAttributes=''  FilterStateMustResolveToSignalObject=off  FilterRTWStateStorageClass=Auto  ParallelPVariant=InternalParameters  IdealPVariant=Disabled  IVariant=InternalParameters  DVariant=InternalParameters  IntegratorVariant=Discrete  SatVariant=Disabled  AWVariant=Passthrough  PCopyVariant=Disabled  TRVariant=Disabled  FdbkBlocksVariant=Forward  IdealPFdbkVariant=Disabled  SatFdbkVariant=Disabled  DerivativeFilterVariant=ForwardEulerFilter  NVariant=InternalParameters  NCopyVariant=Disabled  FilterICVariant=InternalICsFilter  IntegratorICVariant=InternalICs  ExternalResetVariant=Disabled  TRSumVariant=Passthrough  SumFdbkVariant=Disabled  SumVariant=Sum_PID  TsampFilterVariant=InternalTs  TsampNgainVariant=Passthrough  TsampIntegralVariant=Disabled_SignalSpec  ExternalSaturationOutDataTypeStr=Inherit: Same as second input
  Product : Product
  Product1 : Product
  Product2 : Product
  Real-Imag to Complex1 : RealImagToComplex  Commented=on
  Real-Imag to Complex4 : RealImagToComplex
  Scope : Scope  Commented=on  NumInputPorts=2
  Scope1 : Scope
  Scope2 : Scope  NumInputPorts=2
  Scope5 : Scope  NumInputPorts=2
  Scope6 : Scope  NumInputPorts=4
  Signal Specification{1,5..10} (7 alike) : SignalSpecification
  Step : Step  Time=6+20  Before=0.2  After=0.1  SampleTime=0
  Step1 : Step  Time=4.5  Before=1  SampleTime=0
  Switch : Switch  Criteria=u2 > Threshold  Threshold=0.5  SaturateOnIntegerOverflow=off  InputSameDT=off
  Unit Delay : UnitDelay  InitialCondition=1  SampleTime=-1  HasFrameUpgradeWarning=on
  VSM ctrl PQ f : Scope  NumInputPorts=3
  VSM ctrl PQ f1 : Scope  Commented=on  NumInputPorts=4
  VSM_pwm : Scope  NumInputPorts=3
  "[40 60] Hz" : Saturate  UpperLimit=60  LowerLimit=40
  cc_ctrl : Scope  NumInputPorts=3
  dq->abs1 : Subsystem
  dq0 : Scope  Commented=on  NumInputPorts=4
  dq0->abs : Subsystem
  dq0->abs2 : Subsystem
  rPQ : Scope  Commented=on  NumInputPorts=2
  tag scope: Qref=global
  wires:
  Diag/1 -> Bus Selector2/1, Bus Selector6/1, Bus Selector7/1, Bus Selector3/1, Bus Selector9/1, Bus Selector12/1, Bus Selector8/1, Bus Selector1/1, Bus Selector5/1
  Bus Selector7/1 -> VSM_pwm/1  "<pwm>"
  Mux5/1 -> VSM ctrl PQ f/3
  dq0->abs/1(abs) -> Mux5/2  "abs_vc"
  Bus Selector8/1 -> Signal Specification10/1  "<sp_E>"
  Bus Selector11/1 -> Mux6/1  "<sp_i_dq>"
  Bus Selector9/1 -> Bus Selector11/1  "<ccDiag>"
  Bus Selector12/1 -> dq0->abs/1(dq0)  "<vdq>"
  Bus Selector11/3 -> VSM ctrl PQ f1/4, cc_ctrl/3  "<enable_cc>"
  Mux6/1 -> Scope6/2, cc_ctrl/1
  Bus Selector5/1 -> Signal Specification5/1  "<sp_PQ>"
  Bus Selector5/2 -> Signal Specification6/1  "<PQ>"
  Bus Selector5/3 -> Signal Specification7/1  "<sp_f>"
  Bus Selector5/4 -> Signal Specification8/1  "<f>"
  Signal Specification5/1 -> Mux2/1  "PQ_sp"
  Signal Specification7/1 -> Mux3/1  "f_sp"
  Signal Specification8/1 -> VSM ctrl PQ f1/3, Mux3/2  "f_vsm"
  Mux2/1 -> VSM ctrl PQ f/1
  Mux3/1 -> "[40 60] Hz"/1
  Bus Selector1/1 -> Signal Specification9/1  "<f>"
  Signal Specification9/1 -> Mux3/3  "f_pll"
  Signal Specification10/1 -> Mux5/1  "vsm_E_sp"
  Bus Selector11/2 -> dq->abs1/1(dq), Mux6/2  "<i_dq>"
  dq->abs1/1(abs) -> cc_ctrl/2, Scope6/4
  Bus Selector6/1 -> Signal Specification1/1  "<E>"
  Signal Specification1/1 -> Mux5/3  "vsm_E"
  "[40 60] Hz"/1 -> VSM ctrl PQ f/2
  dq0->abs2/1(abs) -> Scope6/1, dq0/4  "|u|"
  Bus Selector3/2 -> VSM_pwm/3, rPQ/2  "<i_out_abc>"
  Bus Selector3/1 -> rPQ/1  "<u_inv_dq>"
  Bus Selector7/2 -> VSM_pwm/2  "<i_inv_abc>"
  Bus Selector2/2 -> dq0->abs2/1(dq0), Demux4/1, dq0/2  "<u_cap_dq0>"
  Real-Imag to Complex4/1 -> Complex to Magnitude-Angle4/1
  Demux4/1 -> Real-Imag to Complex4/1
  Demux4/2 -> Real-Imag to Complex4/2
  Complex to Magnitude-Angle4/1 -> Divide1/1  "cap"
  Signal Specification6/1 -> Demux2/1, VSM ctrl PQ f1/2, Mux2/2  "PQ"
  Bus Selector7/3 -> Divide1/2  "<PQ_out>"
  Demux1/2 -> Real-Imag to Complex1/2
  Demux1/1 -> Real-Imag to Complex1/1
  Real-Imag to Complex1/1 -> Complex to Magnitude-Angle1/1
  Complex to Magnitude-Angle1/2 -> Scope/2  "U_cap"
  Bus Selector2/1 -> Demux1/1, dq0/3, dq0/1  "<u_inv_dq>"
  Demux2/2 -> Add/2
  PID Controller/1 -> [Qref], Scope2/2
  Step/1 -> Add/1, Product/2
  Bus Selector2/4 -> Product/1  "<ENABLED>"
  Add/1 -> Scope2/1, Product1/2
  Product1/1 -> Product2/2, Switch/1
  Step1/1 -> Product1/1
  Abs1/1 -> Compare To Constant1/1
  Compare To Constant1/1 -> Data Type Conversion/1
  Discrete-Time Integrator1/1 -> Scope5/1, Compare To Constant2/1
  Data Type Conversion/1 -> Discrete-Time Integrator1/2, Discrete-Time Integrator1/1
  Compare To Constant2/1 -> Unit Delay/1
  Product2/1 -> PID Controller/1
  Unit Delay/1 -> Switch/2, Scope5/2, Product2/1
  Constant/1 -> Switch/3
  Switch/1 -> Abs1/1, Scope1/1
  Divide1/1 -> Scope/1, Scope6/3

== system AC_base_1_VSM_1_22a/Variant Subsystem3/VSM/Inverter AverageMdl LC SimScape2/Modul F30 fixed DC voltage Average SimScape/ctrlSelect3 ==
  ctrl : Inport
  Bus Creator1 : BusCreator  Inputs=3
  Bus Creator2 : BusCreator  Inputs=3
  Bus Creator3 : BusCreator  Inputs=3
  Bus Selector : BusSelector  OutputSignals=pwm,connect,enable
  Compare To Constant : simulink/Logic and Bit Operations/Compare To Constant  relop=<  const=0.5  OutDataTypeStr=boolean
  Constant : Constant
  Data Type Conversion : DataTypeConversion  OutDataTypeStr=double  SaturateOnIntegerOverflow=off  RndMeth=Floor
  Data Type Conversion1 : DataTypeConversion  OutDataTypeStr=double  SaturateOnIntegerOverflow=off  RndMeth=Floor
  Rate Transition : RateTransition  Integrity=off  Deterministic=off  OutPortSampleTime=0
  Selector1 : Selector  InputPortWidth=3  IndexOptions=Index vector (dialog)  Indices=[1]  OutputSizes=1
  Selector2 : Selector  InputPortWidth=3  IndexOptions=Index vector (dialog)  Indices=2  OutputSizes=1
  Selector3 : Selector  InputPortWidth=3  IndexOptions=Index vector (dialog)  Indices=3  OutputSizes=1
  Sum of Elements : Sum  Inputs=+
  Sum of Elements1 : Sum  Inputs=+  SampleTime=ControlSampleTime
  ctrl1 : Outport  VectorParamsAs1DForOutWhenUnconnected=off
  ctrl2 : Outport  Port=2  VectorParamsAs1DForOutWhenUnconnected=off
  ctrl3 : Outport  Port=3  VectorParamsAs1DForOutWhenUnconnected=off
  wires:
  Rate Transition/1 -> Selector1/1, Selector3/1, Selector2/1
  Selector1/1 -> Bus Creator1/1  "pwm"
  Bus Creator3/1 -> ctrl2/1
  Selector2/1 -> Bus Creator3/1  "pwm"
  Bus Creator1/1 -> ctrl1/1
  ctrl/1 -> Bus Selector/1
  Bus Creator2/1 -> ctrl3/1
  Selector3/1 -> Bus Creator2/1  "pwm"
  Bus Selector/1 -> Rate Transition/1  "<pwm>"
  Data Type Conversion/1 -> Bus Creator1/3, Bus Creator2/3, Bus Creator3/3  "enable"
  Data Type Conversion1/1 -> Bus Creator2/2, Bus Creator3/2, Bus Creator1/2  "connect"
  Constant/1 -> Sum of Elements/1, Sum of Elements1/1
  Bus Selector/2 -> Data Type Conversion1/1  "<connect>"
  Bus Selector/3 -> Compare To Constant/1  "<enable>"
  Compare To Constant/1 -> Data Type Conversion/1

== system AC_base_1_VSM_1_22a/Variant Subsystem3/VSM/Inverter AverageMdl LC SimScape2/Modul F30 fixed DC voltage Average SimScape/measMerge3 ==
  meas1 : Inport
  meas2 : Inport  Port=2
  meas3 : Inport  Port=3
  measMerge123 : Subsystem
  meas : Outport  VectorParamsAs1DForOutWhenUnconnected=off
  wires:
  meas3/1 -> measMerge123/3(meas3)
  meas2/1 -> measMerge123/2(meas2)
  measMerge123/1(meas) -> meas/1
  meas1/1 -> measMerge123/1(meas1)
